simulink model "Full_Model_sim"  (R2022b)
settings: Solver=ode23t  StartTime=0.0  StopTime=1.5  RelTol=1e-3
values from neighbouring files (symbols this model uses):
  Ao = A - L*C    [Observer_Tune.m]
  Bo = [B L]    [Observer_Tune.m]
  Co = eye(3)    [Observer_Tune.m]
  Do = zeros(3, 3)    [Observer_Tune.m]
undefined symbols (not defined in the file or in its folder): bridge, diode, DiscIntNeverNeededParam, Discrete, Gamma, H, J, motor, Phi, pwr, Ri, Rw, sat, Time, uc
libraries: fl_lib x39, nesl_utility x27, ee_lib x25, simulink x3, ctrlSharedLib x1
(part 1 of 3)
settings Model: Creator=gotta  LastModifiedBy=giuliapegoraro
settings SolverCC: MaxConsecutiveMinStep=10  ZeroCrossAlgorithm=Adaptive
settings DataIOCC: Refine=10
settings DebuggingCC: IgnoredZcDiagnostic=none

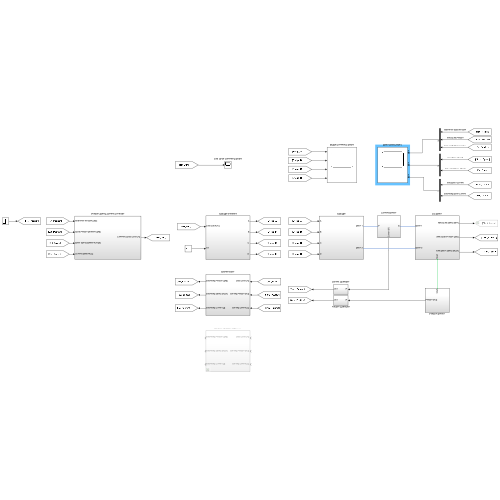
[thumbnail: Simulink's stored preview of the top-level diagram]
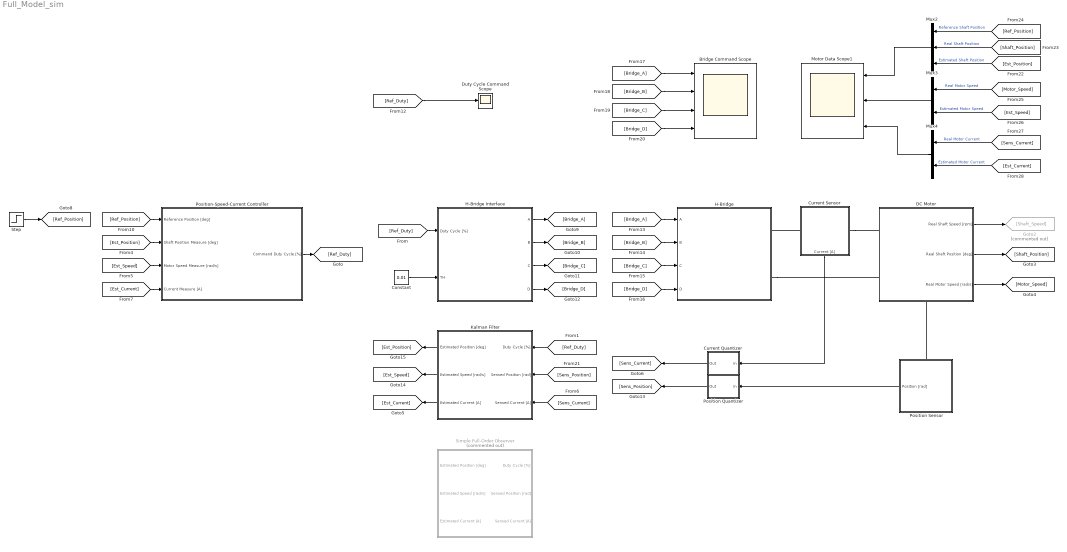
== system Full_Model_sim ==
  Bridge Command Scope : Scope  NumInputPorts=4
  Constant : Constant  Value=0.01
  Current Quantizer : Subsystem
  Current Sensor : Subsystem
      settings: PortSchema="{\"entries\":[{\"content\":{\"sides\":[{\"content\":{\"connectorIds\":[\"Out1\"]},\"type\":\"ConnectorPlacement.EquallySpacedRectSide\",\"uuid\":\"2573d3c3-03c4-452d-9dae-89011d1248da\"},{\"content\":{\"connectorIds\":[],\"side\":\"RIGHT\"},\"type\":\"ConnectorPlacement.EquallySpacedRectSide\",\"uuid\":\"bbe9e370-74cc-46b8-9c24-075015e8eb10\"},{\"content\":{\"connectorIds\":[\"LConn1\"],\"side\":\"TOP\"},\"type\":\"ConnectorPlacement.EquallySpacedRectSide\",\"uuid\":\"b1ce1e52-8e1a-4765-9f85-bff289c8debb\"},{\"content\":{\"connectorIds\":[\"RConn1\"],\"side\":\"BOTTOM\"},\"type\":\"ConnectorPlacement.EquallySpacedRectSide\",\"uuid\":\"0695d450-f3c3-4287-93b9-efed01157391\"}]},\"type\":\"ConnectorPlacement.EquallySpacedConnector\",\"uuid\":\"9343d1eb-a2ec-4ec0-8fde-8976568d4d89\"}],\"packageUris\":[\"http://schema.mathworks.com/mf0/Connector/R2020b\"],\"version\":\"1.0\"}"
  DC Motor : Subsystem
      settings: PortSchema="{\"entries\":[{\"content\":{\"sides\":[{\"content\":{\"connectorIds\":[\"LConn1\",\"LConn2\"]},\"type\":\"ConnectorPlacement.EquallySpacedRectSide\",\"uuid\":\"6ab8a2ca-2e71-4c35-afcd-8b0bd2021176\"},{\"content\":{\"connectorIds\":[\"Out1\",\"Out2\",\"Out3\"],\"side\":\"RIGHT\"},\"type\":\"ConnectorPlacement.EquallySpacedRectSide\",\"uuid\":\"d3dfdd51-7397-4825-b175-78eac32e6d9d\"},{\"content\":{\"connectorIds\":[],\"side\":\"TOP\"},\"type\":\"ConnectorPlacement.EquallySpacedRectSide\",\"uuid\":\"a7cfaff2-0ae6-4fbb-a099-2a304565fee1\"},{\"content\":{\"connectorIds\":[\"RConn1\"],\"side\":\"BOTTOM\"},\"type\":\"ConnectorPlacement.EquallySpacedRectSide\",\"uuid\":\"a0639675-2e22-459b-8bb8-2c2f061728b4\"}]},\"type\":\"ConnectorPlacement.EquallySpacedConnector\",\"uuid\":\"c5b7cd6c-5a44-4892-a55d-8579e461572d\"}],\"packageUris\":[\"http://schema.mathworks.com/mf0/Connector/R2020b\"],\"version\":\"1.0\"}"
  Duty Cycle Command Scope : Scope
  Goto2 : Goto  Commented=on  GotoTag=Shaft_Speed
  H-Bridge : Subsystem
  H-Bridge Interface : Subsystem
  Kalman Filter : Subsystem
  Motor Data Scope1 : Scope  NumInputPorts=3
  Mux2 : Mux  Inputs=3
  Mux3 : Mux  Inputs=2
  Mux4 : Mux  Inputs=2
  Position Quantizer : Subsystem
  Position Sensor : Subsystem
      settings: PortSchema="{\"entries\":[{\"content\":{\"sides\":[{\"content\":{\"connectorIds\":[]},\"type\":\"ConnectorPlacement.EquallySpacedRectSide\",\"uuid\":\"d36fe1c4-850a-4c75-8c52-3756b1598cdf\"},{\"content\":{\"connectorIds\":[\"Out1\"],\"side\":\"RIGHT\"},\"type\":\"ConnectorPlacement.EquallySpacedRectSide\",\"uuid\":\"54a7c68c-1276-40fc-b30e-f6c2515c3006\"},{\"content\":{\"connectorIds\":[\"LConn1\"],\"side\":\"TOP\"},\"type\":\"ConnectorPlacement.EquallySpacedRectSide\",\"uuid\":\"1185fa4c-109a-4ade-aa58-e11090417f23\"}]},\"type\":\"ConnectorPlacement.EquallySpacedConnector\",\"uuid\":\"8f0159e8-c6cb-4893-a3e9-16e7311d52be\"}],\"packageUris\":[\"http://schema.mathworks.com/mf0/Connector/R2020b\"],\"version\":\"1.0\"}"
  Position-Speed-Current Controller : Subsystem
  Simple Full-Order Observer : Subsystem  Commented=on
  Step : Step  Time=0.1  After=170  SampleTime=uc.Ts
  wires:
  DC Motor/3(Real Motor Speed [rad/s]) -> [Motor_Speed]
  Constant/1 -> H-Bridge Interface/2(TH)
  Position-Speed-Current Controller/1(Command Duty Cycle [%]) -> [Ref_Duty]
  [Ref_Duty] -> H-Bridge Interface/1(Duty Cycle [%])
  DC Motor/1(Real Shaft Speed [rpm]) -> Goto2/1
  DC Motor/2(Real Shaft Position [deg]) -> [Shaft_Position]
  Step/1 -> [Ref_Position]
  [Ref_Position] -> Position-Speed-Current Controller/1(Reference Position [deg])
  [Ref_Duty] -> Duty Cycle Command Scope/1
  H-Bridge Interface/1(A) -> [Bridge_A]
  H-Bridge Interface/2(B) -> [Bridge_B]
  H-Bridge Interface/3(C) -> [Bridge_C]
  H-Bridge Interface/4(D) -> [Bridge_D]
  [Bridge_D] -> H-Bridge/4(D)
  [Bridge_C] -> H-Bridge/3(C)
  [Bridge_B] -> H-Bridge/2(B)
  [Bridge_A] -> H-Bridge/1(A)
  [Bridge_A] -> Bridge Command Scope/1
  [Bridge_B] -> Bridge Command Scope/2
  [Bridge_C] -> Bridge Command Scope/3
  [Bridge_D] -> Bridge Command Scope/4
  Position Sensor/1(Position [rad]) -> Position Quantizer/1(In)
  Mux2/1 -> Motor Data Scope1/1
  Mux4/1 -> Motor Data Scope1/3
  Mux3/1 -> Motor Data Scope1/2
  [Ref_Position] -> Mux2/1  "Reference Shaft Position"
  [Shaft_Position] -> Mux2/2  "Real Shaft Position"
  [Est_Position] -> Mux2/3  "Estimated Shaft Position"
  [Motor_Speed] -> Mux3/1  "Real Motor Speed"
  [Est_Speed] -> Mux3/2  "Estimated Motor Speed"
  [Sens_Current] -> Mux4/1  "Real Motor Current"
  [Est_Current] -> Mux4/2  "Estimated Motor Current"
  Current Sensor/1(Current [A]) -> Current Quantizer/1(In)
  [Est_Current] -> Position-Speed-Current Controller/4(Current Measure [A])
  [Est_Position] -> Position-Speed-Current Controller/2(Shaft Position Measure [deg])
  [Est_Speed] -> Position-Speed-Current Controller/3(Motor Speed Measure [rad/s])
  [Ref_Duty] -> Kalman Filter/1(Duty Cycle [%])
  [Sens_Position] -> Kalman Filter/2(Sensed Position [rad])
  [Sens_Current] -> Kalman Filter/3(Sensed Current [A])
  Kalman Filter/1(Estimated Position [deg]) -> [Est_Position]
  Kalman Filter/2(Estimated Speed [rad/s]) -> [Est_Speed]
  Kalman Filter/3(Estimated Current [A]) -> [Est_Current]
  Current Quantizer/1(Out) -> [Sens_Current]
  Position Quantizer/1(Out) -> [Sens_Position]
  connections:
  H-Bridge/RConn2 -- DC Motor/LConn2
  Position Sensor/LConn1 -- DC Motor/RConn1
  Current Sensor/LConn1 -- H-Bridge/RConn1
  Current Sensor/RConn1 -- DC Motor/LConn1

== system Full_Model_sim/Current Quantizer ==
  In : Inport
  Quantizer : Quantizer  QuantizationInterval=INA219.q
  Zero-Order Hold : ZeroOrderHold  Commented=through  SampleTime=uc.Ts
  Out : Outport
  wires:
  Quantizer/1 -> Zero-Order Hold/1
  Zero-Order Hold/1 -> Out/1
  In/1 -> Quantizer/1

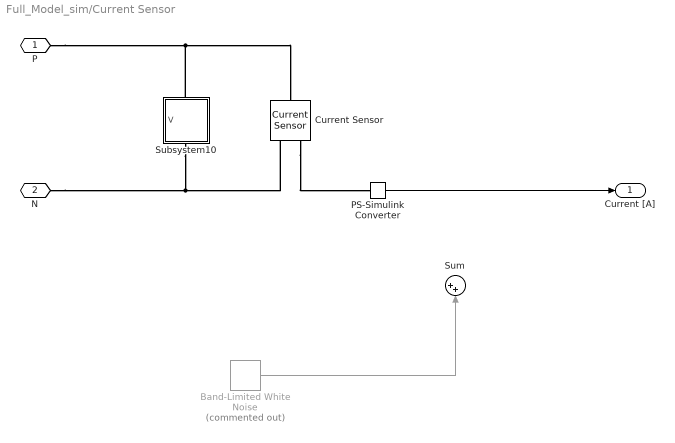
== system Full_Model_sim/Current Sensor ==
  Band-Limited White Noise : simulink/Sources/Band-Limited White Noise  Commented=on  Cov=[0.1]  Ts=0.1  seed=[23341]
  Current Sensor : fl_lib/Electrical/Electrical Sensors/Current Sensor
  PS-Simulink Converter : nesl_utility/PS-Simulink Converter  PhysicalDomain=network_engine_domain  SubClassName=ps_output  LeftPortType=input  RightPortType=output  PseudoPeriodic=off  Frequencies=[]  VectorFormat=inherit  Unit=inherit  AffineConversion=off
  Subsystem10 : Subsystem
      settings: PortSchema="{\"entries\":[{\"content\":{\"sides\":[{\"content\":{\"connectorIds\":[]},\"type\":\"ConnectorPlacement.EquallySpacedRectSide\",\"uuid\":\"2573d3c3-03c4-452d-9dae-89011d1248da\"},{\"content\":{\"connectorIds\":[\"Out1\"],\"side\":\"RIGHT\"},\"type\":\"ConnectorPlacement.EquallySpacedRectSide\",\"uuid\":\"bbe9e370-74cc-46b8-9c24-075015e8eb10\"},{\"content\":{\"connectorIds\":[\"LConn1\"],\"side\":\"TOP\"},\"type\":\"ConnectorPlacement.EquallySpacedRectSide\",\"uuid\":\"b1ce1e52-8e1a-4765-9f85-bff289c8debb\"},{\"content\":{\"connectorIds\":[\"RConn1\"],\"side\":\"BOTTOM\"},\"type\":\"ConnectorPlacement.EquallySpacedRectSide\",\"uuid\":\"0695d450-f3c3-4287-93b9-efed01157391\"}]},\"type\":\"ConnectorPlacement.EquallySpacedConnector\",\"uuid\":\"9343d1eb-a2ec-4ec0-8fde-8976568d4d89\"}],\"packageUris\":[\"http://schema.mathworks.com/mf0/Connector/R2020b\"],\"version\":\"1.0\"}"
  Sum : Sum  Inputs=|++
  P : PMIOPort  Side=Left
  N : PMIOPort  Port=2  Side=Right
  Current [A] : Outport
  wires:
  PS-Simulink Converter/1 -> Current [A]/1
  Band-Limited White Noise/1 -> Sum/2
  connections:
  N/RConn1 -- Subsystem10/RConn1 -- Current Sensor/RConn2
  P/RConn1 -- Subsystem10/LConn1 -- Current Sensor/LConn1
  Current Sensor/RConn1 -- PS-Simulink Converter/LConn1

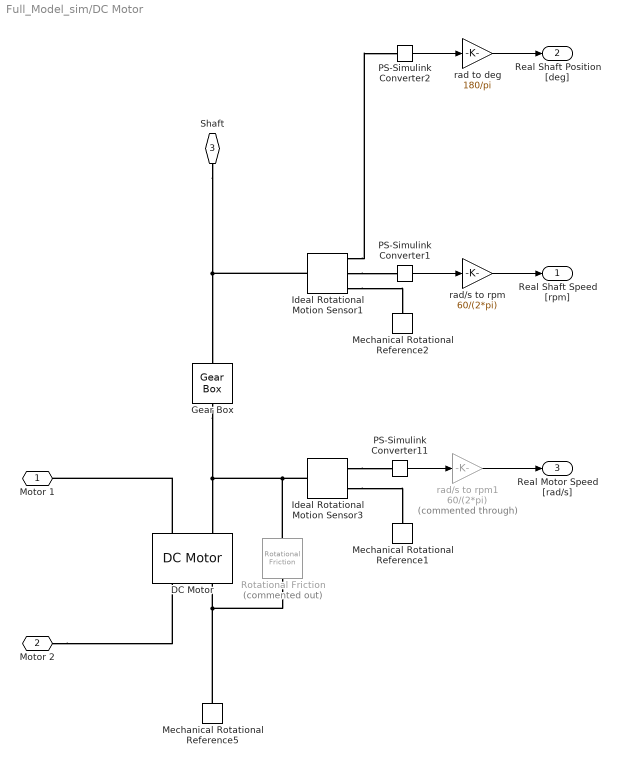
== system Full_Model_sim/DC Motor ==
  DC Motor : ee_lib/Electromechanical/Brushed Motors/DC Motor  field_option=ee.enum.field_option.pm  Rf=100 Ohm  Lf=1 H  Laf=0.15 H  If0=0 A  parameterization=ee.enum.dcparam_option.circuit_param  Ra=motor.Ra Ohm  La=motor.La H  emf_or_torque=ee.enum.emf_or_torque.kv  Kv=motor.Kphi V/(rad/s)  Ki=6.876e-4 N*m/A  T_stall=motor.ts mN*m  w_max=motor.wmo rpm  w_rated=motor.wn rpm  P_rated=0.08 W  V_rated=motor.Vn V  lam_param=ee.enum.lam_param.current  i_noload=motor.Imo A  V_i_noload=motor.Vn V  J=motor.J kg*m^2  lam=motor.B N*m*s/rad  speed0=0 rpm  enable_fault_armature=simscape.enum.onoff.off  rev_faulted=1 / 3  G_faulted_armature=1e-5 S  fault_trigger_armature=ee.enum.faults.faultTrigger.temporal  t_fault_armature=1 s  max_permissible_current_armature=inf A  t_fail_on_current_armature=1 s  enable_fault_field=simscape.enum.onoff.off  G_faulted_field=1e-5 S  fault_trigger_field=ee.enum.faults.faultTrigger.temporal  t_fault_field=1 s  max_permissible_current_field=inf A  t_fail_on_current_field=1 s  fault_action=simscape.enum.assert.action.none  alpha=3.93e-3 1/K  Tmeas=25 degC  thermal_mass=100 J/K  initial_temperature=25 degC
  Gear Box : fl_lib/Mechanical/Mechanisms/Gear Box  ratio=motor.gearbox  t_in_specify=off  t_in_priority=None  t_in=0 N*m  t_in_nominal_specify=off  t_in_nominal_unit=N*m  t_in_nominal_value=1  t_out_specify=off  t_out_priority=None  t_out=0 N*m  t_out_nominal_specify=off  t_out_nominal_unit=N*m  t_out_nominal_value=1
  Ideal Rotational Motion Sensor1 : fl_lib/Mechanical/Mechanical Sensors/Ideal Rotational Motion Sensor  reference=foundation.enum.MeasurementReference.difference  acceleration_port=false  velocity_port=true  position_port=true  wrap_angle=false  offset=0 rad
  Ideal Rotational Motion Sensor3 : fl_lib/Mechanical/Mechanical Sensors/Ideal Rotational Motion Sensor  reference=foundation.enum.MeasurementReference.difference  acceleration_port=false  velocity_port=true  position_port=false  wrap_angle=false  offset=0 rad
      settings: InternalSimscapePortConfiguration="{\"Bottom\":[],\"Left\":[{\"id\":\"R\",\"label\":\"R\",\"type\":\"foundation.mechanical.rotational.rotational\"}],\"Right\":[{\"id\":\"C\",\"label\":\"C\",\"type\":\"foundation.mechanical.rotational.rotational\"},{\"id\":\"W\",\"label\":\"W\",\"type\":\"output\"}],\"Top\":[]}"
  Mechanical Rotational Reference1 : fl_lib/Mechanical/Rotational Elements/Mechanical Rotational Reference
  Mechanical Rotational Reference2 : fl_lib/Mechanical/Rotational Elements/Mechanical Rotational Reference
  Mechanical Rotational Reference5 : fl_lib/Mechanical/Rotational Elements/Mechanical Rotational Reference
  PS-Simulink Converter1 : nesl_utility/PS-Simulink Converter  PhysicalDomain=network_engine_domain  SubClassName=ps_output  LeftPortType=input  RightPortType=output  PseudoPeriodic=off  Frequencies=[]  VectorFormat=inherit  Unit=inherit  AffineConversion=off
  PS-Simulink Converter11 : nesl_utility/PS-Simulink Converter  PhysicalDomain=network_engine_domain  SubClassName=ps_output  LeftPortType=input  RightPortType=output  PseudoPeriodic=off  Frequencies=[]  VectorFormat=inherit  Unit=inherit  AffineConversion=off
  PS-Simulink Converter2 : nesl_utility/PS-Simulink Converter  PhysicalDomain=network_engine_domain  SubClassName=ps_output  LeftPortType=input  RightPortType=output  PseudoPeriodic=off  Frequencies=[]  VectorFormat=inherit  Unit=inherit  AffineConversion=off
  Rotational Friction : fl_lib/Mechanical/Rotational Elements/Rotational Friction  Commented=on  brkwy_trq=25 N*m  brkwy_vel=0.1 rad/s  Col_trq=20 N*m  visc_coef=0.001 N*m*s/rad  w_specify=off  w_priority=None  w=0 rad/s  w_nominal_specify=off  w_nominal_unit=rad/s  w_nominal_value=1  t_specify=off  t_priority=None  t=0 N*m  t_nominal_specify=off  t_nominal_unit=N*m  t_nominal_value=1
  rad to deg : Gain  Gain=180/pi
  rad/s to rpm : Gain  Gain=60/(2*pi)
  rad/s to rpm1 : Gain  Commented=through  Gain=60/(2*pi)
  Motor 1 : PMIOPort  Side=Left
  Motor 2 : PMIOPort  Port=2  Side=Left
  Shaft : PMIOPort  Port=3  Side=Right
  Real Shaft Speed [rpm] : Outport
  Real Shaft Position [deg] : Outport  Port=2
  Real Motor Speed [rad/s] : Outport  Port=3
  wires:
  PS-Simulink Converter11/1 -> rad/s to rpm1/1
  rad/s to rpm/1 -> Real Shaft Speed [rpm]/1
  PS-Simulink Converter1/1 -> rad/s to rpm/1
  rad to deg/1 -> Real Shaft Position [deg]/1
  PS-Simulink Converter2/1 -> rad to deg/1
  rad/s to rpm1/1 -> Real Motor Speed [rad/s]/1
  connections:
  Motor 2/RConn1 -- DC Motor/RConn1
  DC Motor/LConn1 -- Motor 1/RConn1
  Ideal Rotational Motion Sensor3/LConn1 -- Rotational Friction/LConn1 -- DC Motor/LConn2 -- Gear Box/RConn1
  Mechanical Rotational Reference5/LConn1 -- Rotational Friction/RConn1 -- DC Motor/RConn2
  Ideal Rotational Motion Sensor3/RConn1 -- Mechanical Rotational Reference1/LConn1
  Ideal Rotational Motion Sensor3/RConn2 -- PS-Simulink Converter11/LConn1
  Ideal Rotational Motion Sensor1/RConn2 -- PS-Simulink Converter1/LConn1
  Ideal Rotational Motion Sensor1/RConn1 -- Mechanical Rotational Reference2/LConn1
  Ideal Rotational Motion Sensor1/LConn1 -- Gear Box/LConn1 -- Shaft/RConn1
  Ideal Rotational Motion Sensor1/RConn3 -- PS-Simulink Converter2/LConn1
